simulink model "HDLLTE"  (R2017b)
settings: Solver=FixedStepDiscrete  StartTime=0.0  StopTime=simParams.stopTime  RelTol=1e-3
InitFcn:
  | simParams = hdlcoder_lteofdm_modDetectref_init;
  | simParams = hdlcoder_lteofdm_modDetecthdl_init(simParams);
StopFcn:
  | hdlcoder_lteofdm_modDetect_analyze;
undefined symbols (not defined in the file): fft_size
libraries: hdlsllib x29, simulink x22, simulink_need_slupdate x13, dspxfrm3 x2, commchan3 x1, dspmlti4 x1, commrflib2 x1, hdlcodermisc x1, dspsigops x1, dspmathops x1, dspsrcs4 x1
(part 1 of 3)
CloseFcn:
  | if exist('fig', 'var')
  | 
  |     if ishandle(fig.SSS)
  |         close(fig.SSS);
  |     end
  | 
  |     if ishandle(fig.PSS)
  |         close(fig.PSS);
  |     end
  | 
  |     if ishandle(fig.FRQEST)
  |         close(fig.FRQEST);
  |     end
  | 
  |     if ishandle(fig.TX)
  |         close(fig.TX);
  |     end
  | 
  |     if ishandle(fig.Text)
  |         close(fig.Text);
  |     end
  | 
  |     clear CellID correlationOutput;
  |     clear pCellID sCellID PSSpeak PSStimingOffset fig;
  |     clear simLTERxData simLTERxDataValid;
  |     clear simLTETxData simLTETxDataValid;
  |     clear simParams thresholdOut;
  |     clear primaryCellID;
  | 
  | end
settings Model: DataTypeOverride=Off  Creator=The MathWorks, Inc.  LastModifiedBy=trainee
settings DataIOCC: LimitDataPoints=on  SaveFormat=Array  SaveOutput=off  VisualizeSimOutput=off  SaveTime=off
settings OptimizationCC: BlockReduction=off  BooleanDataType=off  ConditionallyExecuteInputs=off  DefaultParameterBehavior=Inlined  LifeSpan=inf
settings DebuggingCC: AlgebraicLoopMsg=error  SaveWithParameterizedLinksMsg=none  UnderspecifiedInitializationDetection=Classic  MergeDetectMultiDrivingBlocksExec=none  SignalResolutionControl=TryResolveAllWithWarning  SingleTaskRateTransMsg=error  ParameterPrecisionLossMsg=none  AllowSymbolicDim=off  StrictBusMsg=ErrorOnBusTreatedAsVector  SFUnexpectedBacktrackingDiag=warning  SFNoUnconditionalDefaultTransitionDiag=warning  SFExecutionAtInitializationDiag=none
settings HardwareCC: ProdBitPerPointer=32  ProdBitPerSizeT=32  ProdBitPerPtrDiffT=32  ProdLargestAtomicFloat=None  ProdIntDivRoundTo=Undefined  ProdEndianess=Unspecified  ProdWordSize=32  ProdHWDeviceType=ASIC/FPGA->ASIC/FPGA  TargetBitPerPointer=64  TargetBitPerSizeT=64  TargetBitPerPtrDiffT=64  TargetLongLongMode=on  TargetIntDivRoundTo=Zero  TargetEndianess=LittleEndian  TargetWordSize=64  TargetHWDeviceType=MATLAB Host  ProdEqTarget=off
settings ModelReferenceCC: PropagateSignalLabelsOutOfModel=off
settings CodeAppCC: StateflowObjectComments=on
settings GRTTargetCC: TargetLangStandard=C89/C90 (ANSI)  GeneratePreprocessorConditionals=Disable all
settings ConfigComp: CovMetricSettings=dw  CovHtmlReporting=on  CovSaveCumulativeToWorkspaceVar=on  CovSaveSingleToWorkspaceVar=on  CovExternalEMLEnable=off  CovSFcnEnable=off

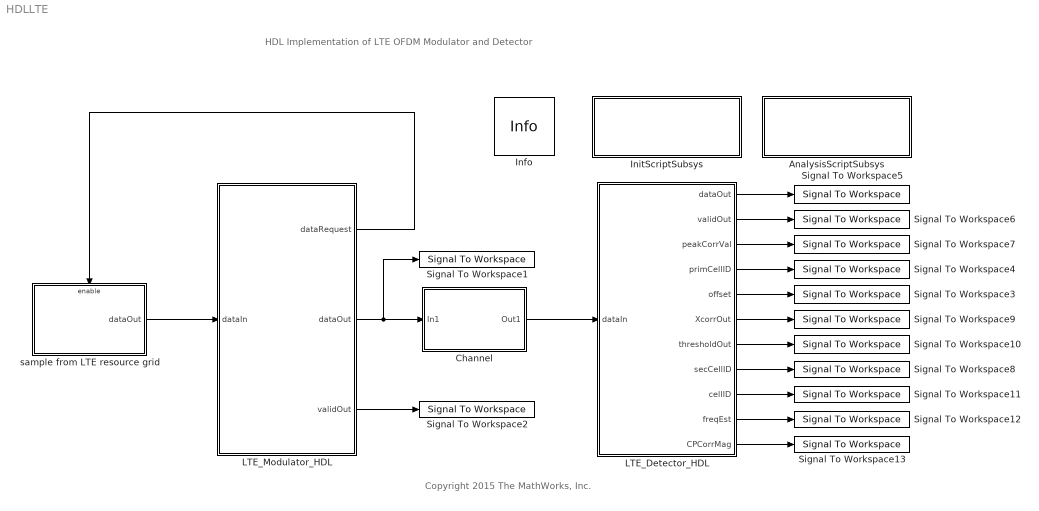
== system HDLLTE ==
  note: HDL Implementation of LTE OFDM Modulator and Detector
  note: Copyright 2015 The MathWorks, Inc.
  AnalysisScriptSubsys : Subsystem
      settings: OpenFcn=edit hdlcoder_lteofdm_modDetect_analyze;
      mask Display: disp('Open post-simulation\n analysis script');
  Channel : Subsystem  mask{timeDelay=simParams.channelDelay, SNR=simParams.channelSNR, gain=simParams.channelGain, frequency=simParams.frequencyOffset}
      mask prompts: timeDelay "Time Delay (samples)"; SNR "SNR (dB)"; gain "Channel Gain"; frequency "Frequency Offset (Hz)"
      mask Display: disp('AWGN &\nFrequency Offset')
  Info : hdlcodermisc/Info  SystemSampleTime=-1
      settings: SourceProductName=HDL Coder  SourceProductBaseCode=HD
  InitScriptSubsys : Subsystem
      settings: OpenFcn=edit hdlcoder_lteofdm_modDetectref_init;
      mask Display: disp('Open LTE initialization\nscript');
  LTE_Detector_HDL : Subsystem
  LTE_Modulator_HDL : Subsystem
  Signal To Workspace1 : SignalToWorkspace  VariableName=simLTETxData
      settings: CopyFcn=dspblkcopystw(gcbh);
  Signal To Workspace10 : SignalToWorkspace  VariableName=thresholdOut
      settings: CopyFcn=dspblkcopystw(gcbh);
  Signal To Workspace11 : SignalToWorkspace  VariableName=cellID
      settings: CopyFcn=dspblkcopystw(gcbh);
  Signal To Workspace12 : SignalToWorkspace  VariableName=freqEst
      settings: CopyFcn=dspblkcopystw(gcbh);
  Signal To Workspace13 : SignalToWorkspace  VariableName=CPCorrMag
      settings: CopyFcn=dspblkcopystw(gcbh);
  Signal To Workspace2 : SignalToWorkspace  VariableName=simLTETxDataValid
      settings: CopyFcn=dspblkcopystw(gcbh);
  Signal To Workspace3 : SignalToWorkspace  VariableName=timingOffset
      settings: CopyFcn=dspblkcopystw(gcbh);
  Signal To Workspace4 : SignalToWorkspace  VariableName=primaryCellID
      settings: CopyFcn=dspblkcopystw(gcbh);
  Signal To Workspace5 : SignalToWorkspace  VariableName=simLTERxData
      settings: CopyFcn=dspblkcopystw(gcbh);
  Signal To Workspace6 : SignalToWorkspace  VariableName=simLTERxDataValid
      settings: CopyFcn=dspblkcopystw(gcbh);
  Signal To Workspace7 : SignalToWorkspace  VariableName=peakCorrelationOutput
      settings: CopyFcn=dspblkcopystw(gcbh);
  Signal To Workspace8 : SignalToWorkspace  VariableName=secondaryCellID
      settings: CopyFcn=dspblkcopystw(gcbh);
  Signal To Workspace9 : SignalToWorkspace  VariableName=correlationOutput
      settings: CopyFcn=dspblkcopystw(gcbh);
  sample from LTE resource grid : Subsystem
  wires:
  LTE_Modulator_HDL/2(dataOut) -> Signal To Workspace1/1, Channel/1(In1)
  LTE_Modulator_HDL/1(dataRequest) -> sample from LTE resource grid/Enable
  sample from LTE resource grid/1(dataOut) -> LTE_Modulator_HDL/1(dataIn)
  LTE_Detector_HDL/1(dataOut) -> Signal To Workspace5/1
  LTE_Detector_HDL/2(validOut) -> Signal To Workspace6/1
  LTE_Detector_HDL/5(offset) -> Signal To Workspace3/1
  LTE_Detector_HDL/7(thresholdOut) -> Signal To Workspace10/1
  LTE_Detector_HDL/6(XcorrOut) -> Signal To Workspace9/1
  LTE_Detector_HDL/3(peakCorrVal) -> Signal To Workspace7/1
  LTE_Detector_HDL/4(primCellID) -> Signal To Workspace4/1
  Channel/1(Out1) -> LTE_Detector_HDL/1(dataIn)
  LTE_Detector_HDL/8(secCellID) -> Signal To Workspace8/1
  LTE_Detector_HDL/9(cellID) -> Signal To Workspace11/1
  LTE_Modulator_HDL/3(validOut) -> Signal To Workspace2/1
  LTE_Detector_HDL/10(freqEst) -> Signal To Workspace12/1
  LTE_Detector_HDL/11(CPCorrMag) -> Signal To Workspace13/1

== system HDLLTE/AnalysisScriptSubsys ==

== system HDLLTE/Channel ==
  In1 : Inport
  ADC : DataTypeConversion  OutDataTypeStr=fixdt(1,16,14)  RndMeth=Nearest
  AWGN : commchan3/AWGN Channel  InputProcessing=Columns as channels (frame based)  seed=67  noiseMode="Signal to noise ratio  (SNR)"  EbNodB=ebno  EsNodB=10  SNRdB=SNR  bitsPerSym=1  Ps=0.0011  Tsym=1  variance=1
  Channel Attenuation : Gain  Gain=gain
  DAC : DataTypeConversion  OutDataTypeStr=double  RndMeth=Nearest
  FIR Decimation : dspmlti4/FIR Decimation  FilterSource=Dialog parameters  h=simParams.hm.*simParams.m  D=simParams.m  filtStruct=Direct form  FilterObject=Hm_firdecim  framing=Allow multirate processing  inputOffset=0  outputBufInitCond=0  roundingMode=Floor  overflowMode=off  firstCoeffDataTypeStr=Inherit: Same word length as input  firstCoeffMin=[]  firstCoeffMax=[]  firstCoeffLastDataTypeStr=Inherit: Same word length as input  outputMin=[]  outputMax=[]
  Phase/ Frequency Offset : commrflib2/Phase// Frequency Offset  phaseOffset=0  freqPort=off  freqOffset=frequency
      settings: SourceProductName=Communications System Toolbox
  Time Delay : Delay  DelayLength=timeDelay  InitialCondition=0
  Out1 : Outport
  wires:
  In1/1 -> DAC/1
  AWGN/1 -> Time Delay/1
  ADC/1 -> Out1/1
  Channel Attenuation/1 -> Phase/ Frequency Offset/1
  Time Delay/1 -> Channel Attenuation/1
  FIR Decimation/1 -> ADC/1
  DAC/1 -> AWGN/1
  Phase/ Frequency Offset/1 -> FIR Decimation/1

== system HDLLTE/InitScriptSubsys ==

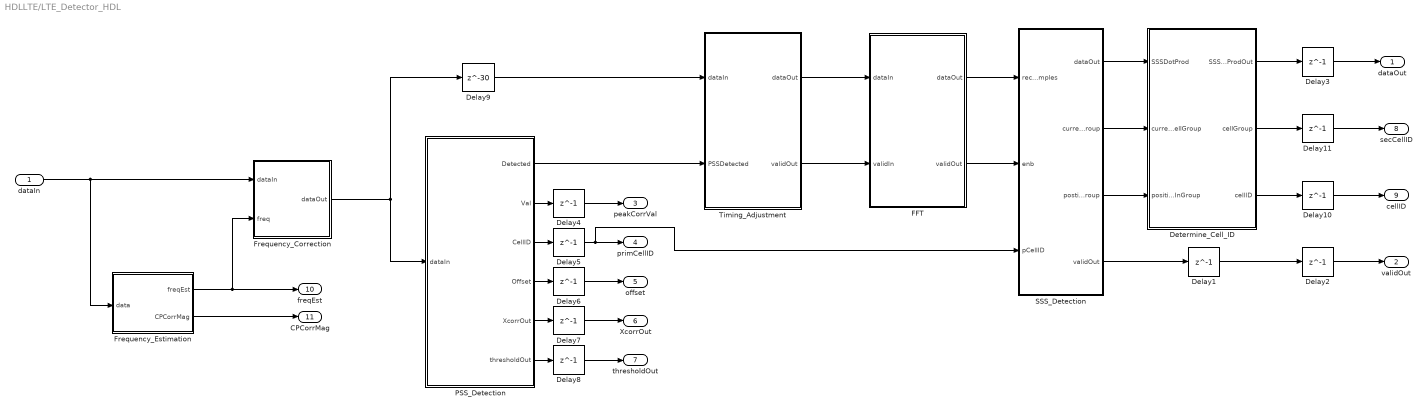
== system HDLLTE/LTE_Detector_HDL ==
  dataIn : Inport
  Delay{1..8,10..11} (10 alike) : Delay  DelayLength=1  InitialCondition=0  UseCircularBuffer=on
  Delay9 : Delay  DelayLength=30  InitialCondition=0  InputProcessing=Columns as channels (frame based)
  Determine_Cell_ID : Subsystem
  FFT : Subsystem
  Frequency_Correction : Subsystem
  Frequency_Estimation : Subsystem
  PSS_Detection : Subsystem
  SSS_Detection : Subsystem
  Timing_Adjustment : Subsystem
  dataOut : Outport
  validOut : Outport  Port=2
  peakCorrVal : Outport  Port=3
  primCellID : Outport  Port=4
  offset : Outport  Port=5
  XcorrOut : Outport  Port=6
  thresholdOut : Outport  Port=7
  secCellID : Outport  Port=8
  cellID : Outport  Port=9
  freqEst : Outport  Port=10
  CPCorrMag : Outport  Port=11
  wires:
  Timing_Adjustment/2(validOut) -> FFT/2(validIn)
  FFT/2(validOut) -> SSS_Detection/2(enb)
  Delay9/1 -> Timing_Adjustment/1(dataIn)
  FFT/1(dataOut) -> SSS_Detection/1(receiveSamples)
  Timing_Adjustment/1(dataOut) -> FFT/1(dataIn)
  SSS_Detection/1(dataOut) -> Determine_Cell_ID/1(SSSDotProd)
  SSS_Detection/2(currentCellGroup) -> Determine_Cell_ID/2(currentCellGroup)
  SSS_Detection/3(postionInGroup) -> Determine_Cell_ID/3(positionInGroup)
  Determine_Cell_ID/1(SSSDotProdOut) -> Delay3/1
  Determine_Cell_ID/2(cellGroup) -> Delay11/1
  Determine_Cell_ID/3(cellID) -> Delay10/1
  SSS_Detection/4(validOut) -> Delay1/1
  Delay1/1 -> Delay2/1
  Delay3/1 -> dataOut/1
  Delay2/1 -> validOut/1
  PSS_Detection/2(Val) -> Delay4/1
  Delay4/1 -> peakCorrVal/1
  PSS_Detection/3(CellID) -> Delay5/1
  Delay5/1 -> SSS_Detection/3(pCellID), primCellID/1
  PSS_Detection/4("Offset ") -> Delay6/1
  Delay6/1 -> offset/1
  PSS_Detection/5(XcorrOut) -> Delay7/1
  Delay7/1 -> XcorrOut/1
  PSS_Detection/6(thresholdOut) -> Delay8/1
  Delay8/1 -> thresholdOut/1
  Delay11/1 -> secCellID/1
  Delay10/1 -> cellID/1
  PSS_Detection/1(Detected) -> Timing_Adjustment/2(PSSDetected)
  dataIn/1 -> Frequency_Estimation/1(data), Frequency_Correction/1(dataIn)
  Frequency_Correction/1(dataOut) -> PSS_Detection/1(dataIn), Delay9/1
  Frequency_Estimation/2(CPCorrMag) -> CPCorrMag/1
  Frequency_Estimation/1(freqEst) -> Frequency_Correction/2(freq), freqEst/1

== system HDLLTE/LTE_Modulator_HDL ==
  dataIn : Inport
  CP_Extension_Windowing : Subsystem
  Delay2 : Delay  DelayLength=1  InitialCondition=0  InputProcessing=Columns as channels (frame based)
  Delay3 : Delay  DelayLength=1
  Delay4 : Delay  DelayLength=1
  Delay5 : Delay
  Delay6 : Delay  DelayLength=1
  FFT_Shift : Subsystem
  Filtering : Subsystem
  IFFT : Subsystem
  OFDM_Symbol_Mapping : Subsystem
  dataRequest : Outport
  dataOut : Outport  Port=2
  validOut : Outport  Port=3
  wires:
  dataIn/1 -> Delay2/1
  OFDM_Symbol_Mapping/1(dataRequest) -> Delay4/1
  OFDM_Symbol_Mapping/3(validOut) -> FFT_Shift/2(validIn)
  OFDM_Symbol_Mapping/2(dataOut) -> FFT_Shift/1(dataIn)
  FFT_Shift/2(validOut) -> IFFT/2(validIn)
  FFT_Shift/1(dataOut) -> IFFT/1(dataIn)
  IFFT/1(dataOut) -> CP_Extension_Windowing/1(dataIn)
  IFFT/2(validOut) -> CP_Extension_Windowing/2(validIn)
  CP_Extension_Windowing/1(dataOut) -> Filtering/1(dataIn)
  Filtering/1(dataOut) -> Delay3/1
  Delay2/1 -> OFDM_Symbol_Mapping/1(dataIn)
  Delay3/1 -> dataOut/1
  Delay4/1 -> dataRequest/1
  CP_Extension_Windowing/2(validOut) -> Delay5/1
  Delay5/1 -> Delay6/1
  Delay6/1 -> validOut/1

== system HDLLTE/sample from LTE resource grid ==
  request1 : EnablePort
  Data Type Conversion : DataTypeConversion  OutDataTypeStr=fixdt(1,16,14)  RndMeth=Nearest
  sample from LTE resource grid : dspsrcs4/Signal From Workspace  X=simParams.LTEGrid(:)  Ts=simParams.TsTx  nsamps=1  OutputAfterFinalValue=Setting to zero  ignoreOrWarnInputAndFrameLengths=off  OutputFrames=on
  dataOut : Outport
  wires:
  Data Type Conversion/1 -> dataOut/1
  sample from LTE resource grid/1 -> Data Type Conversion/1

== system HDLLTE/LTE_Detector_HDL/Determine_Cell_ID ==
  note: N_ID(2)
  note: Calculate detected Cell ID
      | (CellID = 3*N_ID(1) + N_ID(2))
  note: N_ID(1)
  note: If incoming SSS correlation output is greater than that stored in register,
      | store new maximum value, and cell group number, in registers
  note: Store maximum value in register
  note: Store corresponding cell group in register
  SSSDotProd : Inport
  currentCellGroup : Inport  Port=2
  positionInGroup : Inport  Port=3
  Add2 : Sum  OutDataTypeStr=Inherit: Same as first input
  Delay10 : Delay  DelayLength=1  InitialCondition=0  UseCircularBuffer=on
  Gain1 : Gain  Gain=3  OutDataTypeStr=fixdt(0,9,0)
  Relational Operator4 : RelationalOperator  Operator=>  OutDataTypeStr=boolean  RndMeth=Nearest
  Unit Delay Enabled1 : simulink_need_slupdate/Unit Delay Enabled  vinit=0  tsamp=-1
      settings: SourceProductName=Simulink  SourceProductBaseCode=SL
  Unit Delay Enabled3 : simulink_need_slupdate/Unit Delay Enabled  vinit=0  tsamp=-1
      settings: SourceProductName=Simulink  SourceProductBaseCode=SL
  SSSDotProdOut : Outport
  cellGroup : Outport  Port=2
  cellID : Outport  Port=3
  wires:
  Delay10/1 -> SSSDotProdOut/1
  Add2/1 -> cellID/1
  SSSDotProd/1 -> Unit Delay Enabled3/1, Relational Operator4/1, Delay10/1
  positionInGroup/1 -> Add2/2
  Unit Delay Enabled1/1 -> Gain1/1, cellGroup/1
  currentCellGroup/1 -> Unit Delay Enabled1/1
  Relational Operator4/1 -> Unit Delay Enabled3/2, Unit Delay Enabled1/2
  Gain1/1 -> Add2/1
  Unit Delay Enabled3/1 -> Relational Operator4/2

== system HDLLTE/LTE_Detector_HDL/FFT ==
  note: Set input of FFT to input wordlength + FFT growth to allow
      | the output of the FFT to scale. Maximum bit growth is equal
      | to log2(nFFT).
  dataIn : Inport
  validIn : Inport  Port=2
  Data Type Conversion : DataTypeConversion  OutDataTypeStr=fixdt(1,18,10)  RndMeth=Round
  Delay{1..2,4..5} (4 alike) : Delay  DelayLength=1  InitialCondition=0  InputProcessing=Columns as channels (frame based)
  FFT HDL Optimized : dspxfrm3/FFT HDL Optimized  FFTLength=128  Architecture=Streaming Radix 2^2  ComplexMultiplication=Use 3 multipliers and 5 adders  BitReversedOutput=off  BitReversedInput=off  Normalize=off  SimulateUsing=Code generation  RoundingMethod=Floor  ResetInputPort=off  StartOutputPort=off  EndOutputPort=off
      settings: SourceProductName=DSP System Toolbox  SourceProductBaseCode=DS
  Signal Specification : SignalSpecification  Dimensions=1
  Signal Specification1 : SignalSpecification  Dimensions=1
  dataOut : Outport
  validOut : Outport  Port=2
  wires:
  Signal Specification1/1 -> FFT HDL Optimized/2
  Signal Specification/1 -> FFT HDL Optimized/1
  FFT HDL Optimized/2 -> Delay5/1
  FFT HDL Optimized/1 -> Delay4/1
  Delay4/1 -> Data Type Conversion/1
  Delay2/1 -> Signal Specification1/1
  dataIn/1 -> Delay1/1
  validIn/1 -> Delay2/1
  Delay1/1 -> Signal Specification/1
  Data Type Conversion/1 -> dataOut/1
  Delay5/1 -> validOut/1

== system HDLLTE/LTE_Detector_HDL/Frequency_Correction ==
  note: This subsystem corrects the frequency offset using an Numerically Controller Oscillator (NCO) and a conjugate multiplication.
  dataIn : Inport
  freq : Inport  Port=2
  Data Type Conversion : DataTypeConversion  OutDataTypeStr=fixdt(1,16,15)  RndMeth=Nearest
  Delay{1..6} (6 alike) : Delay  DelayLength=1  InitialCondition=0  UseCircularBuffer=on
  Gain : Gain  Gain=2^9  OutDataTypeStr=int16
  NCO HDL Optimized : dspsigops/NCO HDL Optimized  PhaseIncrementSource=Input port  PhaseIncrement=100  PhaseOffsetSource=Property  PhaseOffset=0  DitherSource=Property  NumDitherBits=4  PhaseQuantization=on  NumQuantizerAccumulatorBits=12  LUTCompress=on  ResetAction=off  ValidInputPort=off  Waveform=Complex exponential  PhasePort=off  SimulateUsing=Code generation  AccumulatorWL=16  OutputDataType=Binary point scaling  OutputWL=16  OutputFL=14
      settings: SourceProductName=DSP System Toolbox  SourceProductBaseCode=DS
  Product1 : Product
  Signal Spec : SignalSpecification  Dimensions=1
  Unit Delay Enabled : simulink_need_slupdate/Unit Delay Enabled  vinit=0.0  tsamp=-1
      settings: SourceProductName=Simulink  SourceProductBaseCode=SL
  complexConjugate : Math  Operator=conj  SaturateOnIntegerOverflow=on
  dataOut : Outport
  wires:
  complexConjugate/1 -> Delay3/1
  NCO HDL Optimized/2 -> Unit Delay Enabled/2
  dataIn/1 -> Delay2/1
  Product1/1 -> Delay4/1
  NCO HDL Optimized/1 -> Unit Delay Enabled/1
  Unit Delay Enabled/1 -> complexConjugate/1
  Data Type Conversion/1 -> Delay1/1
  Delay2/1 -> Product1/1
  Delay1/1 -> dataOut/1
  Delay4/1 -> Data Type Conversion/1
  Delay3/1 -> Product1/2
  Gain/1 -> Delay5/1
  freq/1 -> Delay6/1
  Delay6/1 -> Gain/1
  Signal Spec/1 -> NCO HDL Optimized/1
  Delay5/1 -> Signal Spec/1

== system HDLLTE/LTE_Detector_HDL/Frequency_Estimation ==
  data : Inport
  Angle_Filter : Subsystem
  Angle_at_Maximum : Subsystem
  Cyclic_Prefix_Correlator : Subsystem
  Rect_to_Polar : Subsystem
  freqEst : Outport
  CPCorrMag : Outport  Port=2
  wires:
  data/1 -> Cyclic_Prefix_Correlator/1(dataIn)
  Rect_to_Polar/3(validOut) -> Angle_at_Maximum/3(validIn)
  Angle_at_Maximum/1(angleOut) -> Angle_Filter/1(angleIn)
  Rect_to_Polar/2(angleOut) -> Angle_at_Maximum/2(angleIn)
  Rect_to_Polar/1(magOut) -> CPCorrMag/1, Angle_at_Maximum/1(magIn)
  Cyclic_Prefix_Correlator/1(corrOut) -> Rect_to_Polar/1(dataIn)
  Angle_Filter/1(angleOut) -> freqEst/1
  Angle_at_Maximum/2(validOut) -> Angle_Filter/2(en)

== system HDLLTE/LTE_Detector_HDL/PSS_Detection ==
  dataIn : Inport
  Cross_Correlation : Subsystem
  Delay4 : Delay  DelayLength=4  InitialCondition=0  InputProcessing=Columns as channels (frame based)
  Determine_Primary_Cell_ID : Subsystem
  Peak_Detection : Subsystem
  Detected : Outport
  Val : Outport  Port=2
  CellID : Outport  Port=3
  "Offset " : Outport  Port=4
  XcorrOut : Outport  Port=5
  thresholdOut : Outport  Port=6  InitialOutput=0
  wires:
  Determine_Primary_Cell_ID/1(Val) -> Val/1
  Determine_Primary_Cell_ID/2(Cell_ID) -> CellID/1
  Determine_Primary_Cell_ID/4(PSSDetected) -> Detected/1
  Determine_Primary_Cell_ID/3("Offset ") -> "Offset "/1
  Determine_Primary_Cell_ID/5(XcorrOut) -> XcorrOut/1
  Delay4/1 -> thresholdOut/1
  Cross_Correlation/1(PSS0) -> Peak_Detection/1(PSS0)
  Cross_Correlation/2(PSS1) -> Peak_Detection/2(PSS1)
  Cross_Correlation/3(PSS2) -> Peak_Detection/3(PSS2)
  Cross_Correlation/4(Threshold) -> Peak_Detection/4(thresholdIn)
  Peak_Detection/4(PSS0Strength) -> Determine_Primary_Cell_ID/3(PSS0Strength)
  Peak_Detection/12(Xcorr1Out) -> Determine_Primary_Cell_ID/11(Xcorr1In)
  Peak_Detection/7(PSS1Strength) -> Determine_Primary_Cell_ID/6(PSS1Strength)
  Peak_Detection/8(PSS2Detected) -> Determine_Primary_Cell_ID/7(PSS2Detected)
  Peak_Detection/10(PSS2Strength) -> Determine_Primary_Cell_ID/9(PSS2Strength)
  Peak_Detection/2(PSS0Detected) -> Determine_Primary_Cell_ID/1(PSS0Detected)
  Peak_Detection/6(PSS1Offset) -> Determine_Primary_Cell_ID/5(PSS1Offset)
  Peak_Detection/3(PSS0Offset) -> Determine_Primary_Cell_ID/2(PSS0Offset)
  Peak_Detection/9(PSS2Offset) -> Determine_Primary_Cell_ID/8(PSS2Offset)
  Peak_Detection/5(PSS1Detected) -> Determine_Primary_Cell_ID/4(PSS1Detected)
  Peak_Detection/11(Xcorr0Out) -> Determine_Primary_Cell_ID/10(Xcorr0In)
  Peak_Detection/13(Xcorr2Out) -> Determine_Primary_Cell_ID/12(Xcorr2In)
  Peak_Detection/1(thresholdOut) -> Delay4/1
  dataIn/1 -> Cross_Correlation/1(dataIn)

== system HDLLTE/LTE_Detector_HDL/SSS_Detection ==
  receiveSamples : Inport
  enb : Inport  Port=2
  pCellID : Inport  Port=3
  Delay1 : Delay  DelayLength=8  InitialCondition=0  UseCircularBuffer=on
  Delay{2,4..7,9..10} (7 alike) : Delay  DelayLength=1  InitialCondition=0  UseCircularBuffer=on
  Delay11 : Delay  DelayLength=4  InitialCondition=0
  Delay12 : Delay  DelayLength=4  InitialCondition=0
  Delay3 : Delay  InitialCondition=0
  Delay8 : Delay  DelayLength=8  InitialCondition=0  UseCircularBuffer=on
  SSS_Dot_Product : Subsystem
  SSS_Sequence_Update : Subsystem
  Sample_and_Store : Subsystem
  dataOut : Outport
  currentCellGroup : Outport  Port=2
  postionInGroup : Outport  Port=3
  validOut : Outport  Port=4
  wires:
  SSS_Dot_Product/2(SSSDotProd) -> Delay4/1
  SSS_Dot_Product/1(validOut) -> Delay9/1
  Delay3/1 -> SSS_Sequence_Update/3(PositionInGroup)
  Sample_and_Store/3(groupCount) -> SSS_Sequence_Update/2(cellGroup)
  Delay2/1 -> Delay3/1
  enb/1 -> Delay6/1
  receiveSamples/1 -> Delay7/1
  pCellID/1 -> Delay2/1
  Sample_and_Store/2(validOut) -> SSS_Sequence_Update/1(validIn)
  Delay7/1 -> Sample_and_Store/1(samplesIn)
  Delay6/1 -> Sample_and_Store/2(enb)
  Sample_and_Store/1(dataOut) -> Delay12/1
  SSS_Sequence_Update/1(validOut) -> SSS_Dot_Product/2(validIn)
  SSS_Sequence_Update/2(seqOut) -> SSS_Dot_Product/3(seqIn)
  SSS_Sequence_Update/3(endofGroup) -> SSS_Dot_Product/4(reset)
  SSS_Sequence_Update/4(detectedPSS) -> Delay8/1
  Delay8/1 -> Delay10/1
  Delay1/1 -> Delay5/1
  Delay10/1 -> postionInGroup/1
  Delay5/1 -> currentCellGroup/1
  Delay4/1 -> dataOut/1
  Delay9/1 -> validOut/1
  Sample_and_Store/4(currentCellGroup) -> Delay11/1
  Delay11/1 -> Delay1/1
  Delay12/1 -> SSS_Dot_Product/1(dataIn)

== system HDLLTE/LTE_Detector_HDL/Timing_Adjustment ==
  note: Detect PSS detection strobe, and create
      | valid high signal.
  note: Delay signal so that once the PSS
      | has been detected, the resource block
      | containing the SSS signal (the previous
      | block) is aligned here.
  note: Only output samples once
      | the detected strobe has
      | been received.
  note: PSS detect strobe is high at the end of the PSS
      | sequence, so delay must be for the full 128 samples
      | of the PSS, and the full 128 samples of the SSS, plus
      | a single short CP length of 9 samples for 128-point
      | FFT.
  dataIn : Inport
  PSSDetected : Inport  Port=2
  Constant : Constant  Value=complex(0)  OutDataTypeStr=fixdt(1,16,15)  SampleTime=simParams.TsRx
  Constant1 : Constant  OutDataTypeStr=boolean  SampleTime=simParams.TsRx
  Delay1 : Delay  DelayLength=265  InitialCondition=0  InputProcessing=Columns as channels (frame based)
  Delay{2..5} (4 alike) : Delay  DelayLength=1  InitialCondition=0  UseCircularBuffer=on
  Switch : Switch  Criteria=u2 > Threshold
  Unit Delay Enabled1 : simulink_need_slupdate/Unit Delay Enabled  vinit=0.0  tsamp=-1
      settings: SourceProductName=Simulink  SourceProductBaseCode=SL
  dataOut : Outport
  validOut : Outport  Port=2
  wires:
  Delay5/1 -> validOut/1
  Delay4/1 -> dataOut/1
  Delay3/1 -> Delay1/1
  Delay2/1 -> Unit Delay Enabled1/2
  Constant/1 -> Switch/3
  Delay1/1 -> Switch/1
  dataIn/1 -> Delay3/1
  Switch/1 -> Delay4/1
  PSSDetected/1 -> Delay2/1
  Unit Delay Enabled1/1 -> Switch/2, Delay5/1
  Constant1/1 -> Unit Delay Enabled1/1

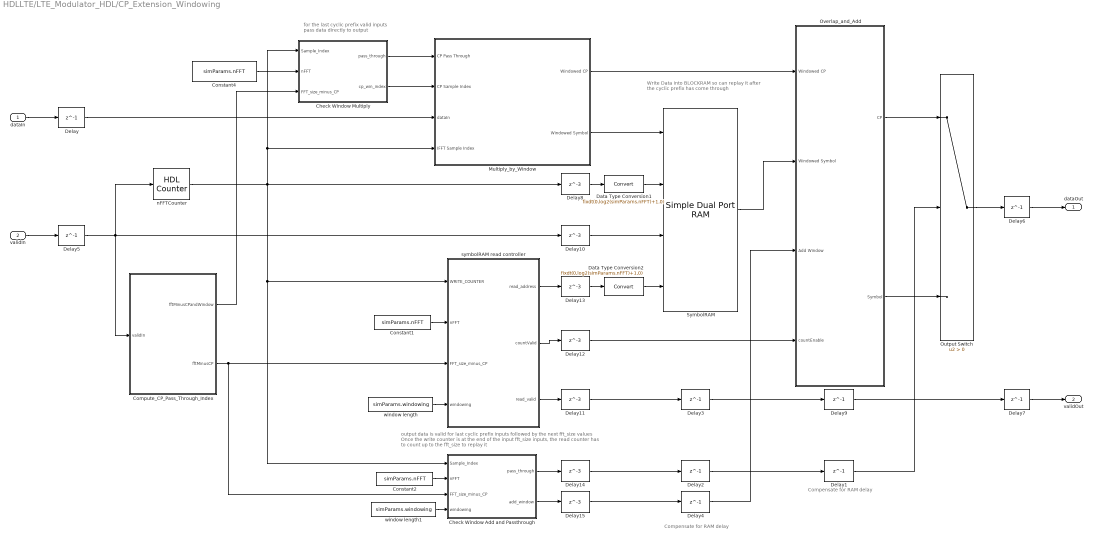
== system HDLLTE/LTE_Modulator_HDL/CP_Extension_Windowing ==
  note: Compensate for RAM delay
  note: output data is valid for last cyclic prefix inputs followed by the next fft_size values
      | Once the write counter is at the end of the input fft_size inputs,
      | the read counter has to count up to the fft_size to replay it
  note: Write Data into BLOCKRAM so can
      | replay it after the cyclic prefix has come through
  note: for the last cyclic prefix valid inputs
      | pass data directly to output
  note: Compensate for RAM delay
  dataIn : Inport
  validIn : Inport  Port=2
  Check Window Add and Passthrough : MATLAB Function  TreatAsAtomicUnit=on
  "Check Window Multiply " : MATLAB Function  TreatAsAtomicUnit=on
  Compute_CP_Pass_Through_Index : Subsystem
  Constant1 : Constant  Value=simParams.nFFT  VectorParams1D=off  OutDataTypeStr=uint16  SampleTime=simParams.TsTx
  Constant2 : Constant  Value=simParams.nFFT  VectorParams1D=off  OutDataTypeStr=uint16  SampleTime=simParams.TsTx
  Constant4 : Constant  Value=simParams.nFFT  VectorParams1D=off  OutDataTypeStr=uint16  SampleTime=simParams.TsTx
  Data Type Conversion1 : DataTypeConversion  OutDataTypeStr=fixdt(0,log2(simParams.nFFT)+1,0)
  Data Type Conversion2 : DataTypeConversion  OutDataTypeStr=fixdt(0,log2(simParams.nFFT)+1,0)
  Delay{,5..7} (4 alike) : Delay  DelayLength=1
  Delay1 : Delay  DelayLength=1  InitialCondition=0  UseCircularBuffer=on
  Delay{8,10..15} (7 alike) : Delay  DelayLength=3  InitialCondition=0  InputProcessing=Columns as channels (frame based)
  Delay2 : Delay  DelayLength=1  InitialCondition=0  InputProcessing=Columns as channels (frame based)
  Delay3 : Delay  DelayLength=1  InitialCondition=0  InputProcessing=Columns as channels (frame based)
  Delay4 : Delay  DelayLength=1  InitialCondition=0  InputProcessing=Columns as channels (frame based)
  Delay9 : Delay  DelayLength=1  InitialCondition=0  UseCircularBuffer=on
  Multiply_by_Window : Subsystem
  Output Switch : Switch  Criteria=u2 > Threshold
  Overlap_and_Add : Subsystem
  SymbolRAM : hdlsllib/HDL RAMs/Simple Dual Port RAM  ram_size=log2(simParams.nFFT)+1
      settings: SourceProductName=HDL Coder  SourceProductBaseCode=HD
  nFFTCounter : hdlsllib/Sources/HDL Counter  CountType=Count limited  CountInit=0  CountStep=1  CountMax=simParams.nFFT-1  CountFromType=Initial value  CountFrom=0  CountResetPort=off  CountLoadPort=off  CountEnbPort=on  CountDirPort=off  CountDataType=Unsigned  CountWordLen=log2(simParams.nFFT)  CountFracLen=0  CountSampTime=1
      settings: SourceProductBaseCode=HD
  symbolRAM read controller : MATLAB Function  TreatAsAtomicUnit=on
  window length : Constant  Value=simParams.windowing  OutDataTypeStr=uint16  SampleTime=simParams.TsTx
  window length1 : Constant  Value=simParams.windowing  OutDataTypeStr=uint16  SampleTime=simParams.TsTx
  dataOut : Outport
  validOut : Outport  Port=2
  wires:
  Data Type Conversion1/1 -> SymbolRAM/2
  Data Type Conversion2/1 -> SymbolRAM/4
  "Check Window Multiply "/1(pass_through) -> Multiply_by_Window/1(CP Pass Through)
  Output Switch/1 -> Delay6/1
  symbolRAM read controller/1(read_address) -> Delay13/1
  Compute_CP_Pass_Through_Index/1(fftMinusCPandWindow) -> "Check Window Multiply "/3(FFT_size_minus_CP)
  validIn/1 -> Delay5/1
  "Check Window Multiply "/2(cp_win_index) -> Multiply_by_Window/2(CP Sample Index)
  dataIn/1 -> Delay/1
  Multiply_by_Window/2(Windowed Symbol) -> SymbolRAM/1
  Compute_CP_Pass_Through_Index/2(fftMinusCP) -> Check Window Add and Passthrough/3(FFT_size_minus_CP), symbolRAM read controller/3(FFT_size_minus_CP)
  SymbolRAM/1 -> Overlap_and_Add/2(Windowed Symbol)
  Delay4/1 -> Overlap_and_Add/3(Add Window)
  Overlap_and_Add/2(Symbol) -> Output Switch/3
  Delay3/1 -> Delay9/1
  Delay9/1 -> Delay7/1
  Delay2/1 -> Delay1/1
  Delay1/1 -> Output Switch/2
  Multiply_by_Window/1(Windowed CP) -> Overlap_and_Add/1(Windowed CP)
  Delay/1 -> Multiply_by_Window/3(dataIn)
  Delay6/1 -> dataOut/1
  Delay7/1 -> validOut/1
  nFFTCounter/1 -> "Check Window Multiply "/1(Sample_Index), Multiply_by_Window/4(IFFT Sample Index), Delay8/1, Check Window Add and Passthrough/1(Sample_Index), symbolRAM read controller/1(WRITE_COUNTER)
  Delay5/1 -> nFFTCounter/1, Compute_CP_Pass_Through_Index/1(validIn), Delay10/1
  symbolRAM read controller/2(countValid) -> Delay12/1
  symbolRAM read controller/3(read_valid) -> Delay11/1
  Check Window Add and Passthrough/1(pass_through) -> Delay14/1
  Check Window Add and Passthrough/2(add_window) -> Delay15/1
  Overlap_and_Add/1(CP) -> Output Switch/1
  Delay8/1 -> Data Type Conversion1/1
  Delay10/1 -> SymbolRAM/3
  Delay12/1 -> Overlap_and_Add/4(countEnable)
  Delay11/1 -> Delay3/1
  Delay13/1 -> Data Type Conversion2/1
  Delay14/1 -> Delay2/1
  Delay15/1 -> Delay4/1
  Constant4/1 -> "Check Window Multiply "/2(nFFT)
  Constant1/1 -> symbolRAM read controller/2(nFFT)
  window length/1 -> symbolRAM read controller/4(windowing)
  window length1/1 -> Check Window Add and Passthrough/4(windowing)
  Constant2/1 -> Check Window Add and Passthrough/2(nFFT)

== system HDLLTE/LTE_Modulator_HDL/FFT_Shift ==
  note: Count 2 full FFT frames
  note: If a full IFFT frame OR 2 full FFT frames have been counted and written into RAM, enable reading from RAM.
  note: Compensate for RAM latency
  dataIn : Inport
  validIn : Inport  Port=2
  " " : simulink/Logic and Bit Operations/Compare To Constant  relop===  const=2*simParams.nFFT-1  OutDataTypeStr=boolean
  " " : simulink/Logic and Bit Operations/Compare To Constant  relop===  const=simParams.nFFT-1  OutDataTypeStr=boolean
  Compute_Read_Address : Subsystem
  Data Type Conversion : DataTypeConversion  OutDataTypeStr=fixdt(0,log2(simParams.nFFT)+1,0)
  Data Type Conversion1 : DataTypeConversion  OutDataTypeStr=fixdt(0,log2(simParams.nFFT)+1,0)
  Delay{,1..4} (5 alike) : Delay  DelayLength=1
  Dual Port RAM : hdlsllib/HDL RAMs/Dual Port RAM  ram_size=log2(simParams.nFFT)+1
      settings: SourceProductName=HDL Coder  SourceProductBaseCode=HD
  HDL Counter : hdlsllib/Sources/HDL Counter  CountType=Count limited  CountInit=0  CountStep=1  CountMax=simParams.nFFT*2-1  CountFromType=Initial value  CountFrom=0  CountResetPort=off  CountLoadPort=off  CountEnbPort=on  CountDirPort=off  CountDataType=Unsigned  CountWordLen=log2(simParams.nFFT)+1  CountFracLen=0  CountSampTime=1
      settings: SourceProductBaseCode=HD
  Logical Operator : Logic  Operator=OR  IconShape=distinctive  AllPortsSameDT=off  OutDataTypeStr=boolean
  Terminator : Terminator
  dataOut : Outport
  validOut : Outport  Port=2
  wires:
  validIn/1 -> Delay3/1
  HDL Counter/1 -> " "/1, " "/1, Data Type Conversion/1
  dataIn/1 -> Delay4/1
  Data Type Conversion1/1 -> Dual Port RAM/4
  Data Type Conversion/1 -> Dual Port RAM/2
  Dual Port RAM/1 -> Terminator/1
  " "/1 -> Logical Operator/1
  " "/1 -> Logical Operator/2
  Dual Port RAM/2 -> Delay2/1
  Logical Operator/1 -> Compute_Read_Address/1(rdEnable)
  Compute_Read_Address/1(rdAddr) -> Data Type Conversion1/1
  Compute_Read_Address/2(rdValid) -> Delay/1
  Delay/1 -> Delay1/1
  Delay1/1 -> validOut/1
  Delay2/1 -> dataOut/1
  Delay3/1 -> Dual Port RAM/3, HDL Counter/1
  Delay4/1 -> Dual Port RAM/1

== system HDLLTE/LTE_Modulator_HDL/Filtering ==
  dataIn : Inport
  Delay : Delay  DelayLength=1
  Delay3 : Delay  DelayLength=1
  Filter1 : DiscreteFir  Tag=BlockMethodSubSystem  FilterStructure=Direct form symmetric  Coefficients=simParams.h  OutDataTypeStr=Inherit: Same as input
  dataOut : Outport
  wires:
  dataIn/1 -> Delay/1
  Delay/1 -> Filter1/1
  Delay3/1 -> dataOut/1
  Filter1/1 -> Delay3/1

== system HDLLTE/LTE_Modulator_HDL/IFFT ==
  note: Set input of FFT to input wordlength + FFT growth to allow
      | the output of the FFT to scale. Maximum bit growth is equal
      | to log2(nFFT).
  dataIn : Inport
  validIn : Inport  Port=2
  Data Type Conversion : DataTypeConversion  OutDataTypeStr=fixdt(1,23,21)  RndMeth=Nearest
  Delay{1..2,4..5} (4 alike) : Delay  DelayLength=1  InitialCondition=0  InputProcessing=Columns as channels (frame based)
  IFFT HDL Optimized : dspxfrm3/IFFT HDL Optimized  FFTLength=simParams.nFFT  Architecture=Streaming Radix 2^2  ComplexMultiplication=Use 3 multipliers and 5 adders  BitReversedOutput=off  BitReversedInput=off  Normalize=on  SimulateUsing=Code generation  RoundingMethod=Floor  ResetInputPort=off  StartOutputPort=off  EndOutputPort=off
      settings: SourceProductName=DSP System Toolbox  SourceProductBaseCode=DS
  Signal Specification : SignalSpecification  Dimensions=1
  Signal Specification1 : SignalSpecification  Dimensions=1
  dataOut : Outport
  validOut : Outport  Port=2
  wires:
  validIn/1 -> Delay2/1
  dataIn/1 -> Delay1/1
  Delay4/1 -> dataOut/1
  Delay5/1 -> validOut/1
  Delay1/1 -> Data Type Conversion/1
  Delay2/1 -> Signal Specification1/1
  IFFT HDL Optimized/1 -> Delay4/1
  IFFT HDL Optimized/2 -> Delay5/1
  Signal Specification/1 -> IFFT HDL Optimized/1
  Signal Specification1/1 -> IFFT HDL Optimized/2
  Data Type Conversion/1 -> Signal Specification/1

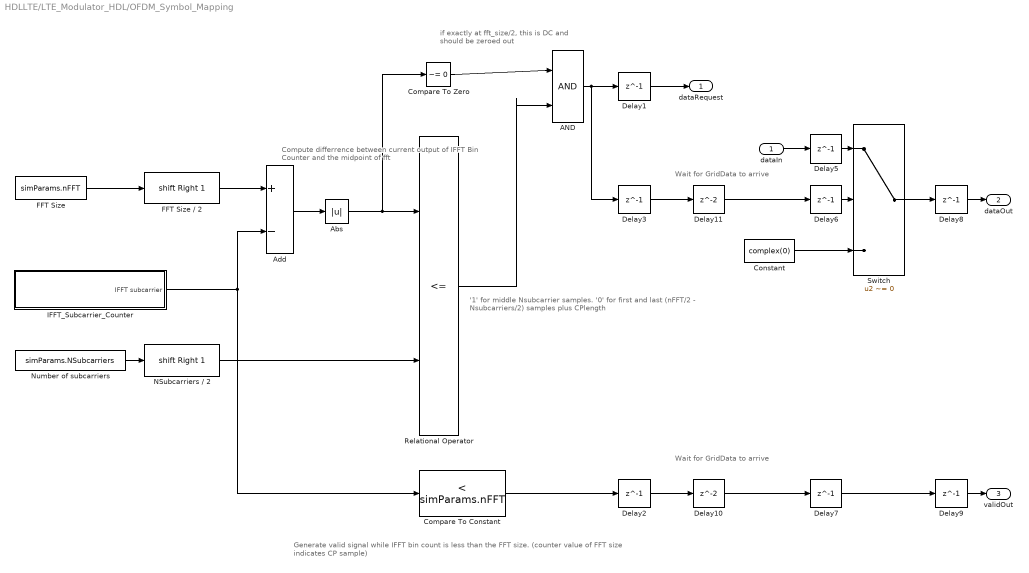
== system HDLLTE/LTE_Modulator_HDL/OFDM_Symbol_Mapping ==
  note: Wait for GridData to
      | arrive
  note: Generate valid signal while IFFT bin count is less than the FFT size.
      | (counter value of FFT size indicates CP sample)
  note: Compute differrence between current output of IFFT Bin Counter and the midpoint of fft
  note: if exactly at fft_size/2, this is DC
      | and should be zeroed out
  note: '1' for middle Nsubcarrier samples.
      | '0' for first and last (nFFT/2 - Nsubcarriers/2) samples
      | plus CPlength
  note: Wait for GridData to
      | arrive
  dataIn : Inport
  AND : Logic  IconShape=distinctive  AllPortsSameDT=off  OutDataTypeStr=boolean
  Abs : Abs
  Add : Sum  Inputs=+-  OutDataTypeStr=fixdt(1,16,0)
  Compare To Constant : simulink/Logic and Bit Operations/Compare To Constant  relop=<  const=simParams.nFFT  OutDataTypeStr=boolean
  Compare To Zero : simulink/Logic and Bit Operations/Compare To Zero  relop=~=  OutDataTypeStr=boolean
  Constant : Constant  Value=complex(0)  OutDataTypeStr=fixdt(1,16,14)  SampleTime=simParams.TsTx
  Delay{1..3,5..9} (8 alike) : Delay  DelayLength=1  InitialCondition=0  InputProcessing=Columns as channels (frame based)
  Delay10 : Delay  InitialCondition=0  InputProcessing=Columns as channels (frame based)
  Delay11 : Delay  InitialCondition=0  InputProcessing=Columns as channels (frame based)
  FFT Size : Constant  Value=simParams.nFFT  OutDataTypeStr=fixdt(0,ceil(log2(simParams.nFFT))+1,0)  SampleTime=simParams.TsTx
  FFT Size / 2 : ArithShift  BitShiftNumber=1  BitShiftDirection=Right
  IFFT_Subcarrier_Counter : Subsystem
  NSubcarriers / 2 : ArithShift  BitShiftNumber=1  BitShiftDirection=Right
  Number of subcarriers : Constant  Value=simParams.NSubcarriers  OutDataTypeStr=fixdt(0,12,0)  SampleTime=simParams.TsTx
  Relational Operator : RelationalOperator  Operator=<=  OutDataTypeStr=boolean  RndMeth=Nearest
  Switch : Switch  Criteria=u2 ~= 0
  dataRequest : Outport
  dataOut : Outport  Port=2
  validOut : Outport  Port=3
  wires:
  Compare To Zero/1 -> AND/1
  Compare To Constant/1 -> Delay2/1
  dataIn/1 -> Delay5/1
  AND/1 -> Delay3/1, Delay1/1
  IFFT_Subcarrier_Counter/1(IFFT subcarrier) -> Add/2, Compare To Constant/1
  FFT Size/1 -> FFT Size / 2/1
  Abs/1 -> Compare To Zero/1, Relational Operator/1
  NSubcarriers / 2/1 -> Relational Operator/2
  Add/1 -> Abs/1
  FFT Size / 2/1 -> Add/1
  Switch/1 -> Delay8/1
  Relational Operator/1 -> AND/2
  Delay2/1 -> Delay10/1
  Delay3/1 -> Delay11/1
  Delay5/1 -> Switch/1
  Constant/1 -> Switch/3
  Delay7/1 -> Delay9/1
  Delay8/1 -> dataOut/1
  Delay9/1 -> validOut/1
  Delay10/1 -> Delay7/1
  Delay11/1 -> Delay6/1
  Delay6/1 -> Switch/2
  Delay1/1 -> dataRequest/1
  Number of subcarriers/1 -> NSubcarriers / 2/1

== system HDLLTE/LTE_Detector_HDL/Frequency_Estimation/Angle_Filter ==
  note: This subsystem implements a 1-pole IIR filter to perform further averaging of the correlation angle results. The filter's gain is normalized to 0dB and an efficient implementation which requires only 1 multiplier is used.
  angleIn : Inport
  en : Inport  Port=2
  Add : Sum  Inputs=|-+
  Add1 : Sum  Inputs=|-+
  Delay1 : Delay  DelayLength=1  InitialCondition=0  UseCircularBuffer=on
  Delay2 : Delay  DelayLength=1  InitialCondition=0  UseCircularBuffer=on
  Delay3 : Delay  DelayLength=1  InitialCondition=0  UseCircularBuffer=on
  Gain : Gain  Gain=2^-2  OutDataTypeStr=Inherit: Same as input
  Unit Delay Enabled : simulink_need_slupdate/Unit Delay Enabled  vinit=0.0  tsamp=-1
      settings: SourceProductName=Simulink  SourceProductBaseCode=SL
  angleOut : Outport
  wires:
  angleIn/1 -> Delay2/1
  Add/1 -> Gain/1
  Gain/1 -> Add1/1
  Unit Delay Enabled/1 -> Add/2, Add1/2, Delay1/1
  Add1/1 -> Unit Delay Enabled/1
  en/1 -> Delay3/1
  Delay1/1 -> angleOut/1
  Delay2/1 -> Add/1
  Delay3/1 -> Unit Delay Enabled/2

== system HDLLTE/LTE_Detector_HDL/Frequency_Estimation/Angle_at_Maximum ==
  note: This subsystem records the maximum CP correlation level, and the corresponding phase angle of the result, across windows of time equivalent to 1 slot (960 samples). A counter is used to reset the running max and record the final phase value, which is then passed to the output and qualified by the validOut signal.
  note: Store current mag & angle if mag is greater than previous max mag.
  note: This register stores the current running max magnitude in the current time window
  magIn : Inport
  angleIn : Inport  Port=2
  validIn : Inport  Port=3
  Compare To Constant : simulink/Logic and Bit Operations/Compare To Constant  relop===  const=0  OutDataTypeStr=boolean
  Delay{1..3,5} (4 alike) : Delay  DelayLength=1  InitialCondition=0  UseCircularBuffer=on
  HDL Counter : hdlsllib/Sources/HDL Counter  CountType=Count limited  CountInit=0  CountStep=1  CountMax=959  CountFromType=Initial value  CountFrom=0  CountResetPort=off  CountLoadPort=off  CountEnbPort=on  CountDirPort=off  CountDataType=Unsigned  CountWordLen=10  CountFracLen=0  CountSampTime=1
      settings: SourceProductBaseCode=HD
  Logical Operator : Logic  Operator=OR  IconShape=distinctive  AllPortsSameDT=off  OutDataTypeStr=boolean
  Relational Operator : RelationalOperator  Operator=>  OutDataTypeStr=boolean  RndMeth=Nearest
  Unit Delay Enabled : simulink_need_slupdate/Unit Delay Enabled  vinit=0.0  tsamp=-1
      settings: SourceProductName=Simulink  SourceProductBaseCode=SL
  Unit Delay Enabled1 : simulink_need_slupdate/Unit Delay Enabled  vinit=0.0  tsamp=-1
      settings: SourceProductName=Simulink  SourceProductBaseCode=SL
  Unit Delay Enabled2 : simulink_need_slupdate/Unit Delay Enabled  vinit=0.0  tsamp=-1
      settings: SourceProductName=Simulink  SourceProductBaseCode=SL
  angleOut : Outport
  validOut : Outport  Port=2
  wires:
  magIn/1 -> Delay5/1
  angleIn/1 -> Delay1/1
  HDL Counter/1 -> Compare To Constant/1
  Compare To Constant/1 -> Unit Delay Enabled2/2, Logical Operator/2, Delay3/1
  Unit Delay Enabled1/1 -> Unit Delay Enabled2/1
  validIn/1 -> Delay2/1
  Delay5/1 -> Relational Operator/1, Unit Delay Enabled/1
  Delay2/1 -> HDL Counter/1
  Unit Delay Enabled2/1 -> angleOut/1
  Delay3/1 -> validOut/1
  Unit Delay Enabled/1 -> Relational Operator/2
  Relational Operator/1 -> Logical Operator/1
  Logical Operator/1 -> Unit Delay Enabled1/2, Unit Delay Enabled/2
  Delay1/1 -> Unit Delay Enabled1/1

== system HDLLTE/LTE_Detector_HDL/Frequency_Estimation/Cyclic_Prefix_Correlator ==
  note: Correlate the signal with itself
      | delayed by the FFT length (128 samples).
  note: Integrate across part of the CP length, which is 9 samples. However we use 8 samples here to optimize for HDL implementation.
  note: Finally average across 7 OFDM symbols, i.e. the number in
      | each slot.
  dataIn : Inport
  Delay1 : Delay  DelayLength=1  InitialCondition=0  UseCircularBuffer=on
  Delay2 : Delay  DelayLength=128  InitialCondition=0
  Delay3 : Delay  DelayLength=1  InitialCondition=0  UseCircularBuffer=on
  Delay5 : Delay  DelayLength=1  InitialCondition=0  UseCircularBuffer=on
  Moving_Average : Subsystem
  Product : Product  OutDataTypeStr=fixdt(1,24,23)  RndMeth=Round
  Slot_Average : Subsystem
  complexConj : Math  Operator=conj  SaturateOnIntegerOverflow=on
  corrOut : Outport
  wires:
  Product/1 -> Delay5/1
  Delay3/1 -> Product/2
  Delay2/1 -> complexConj/1
  Slot_Average/1(dataOut) -> corrOut/1
  Moving_Average/1(dataOut) -> Slot_Average/1(dataIn)
  complexConj/1 -> Delay3/1
  Delay5/1 -> Moving_Average/1(dataIn)
  Delay1/1 -> Product/1
  dataIn/1 -> Delay2/1, Delay1/1

== system HDLLTE/LTE_Detector_HDL/Frequency_Estimation/Rect_to_Polar ==
  dataIn : Inport
  Complex to Magnitude-Angle HDL Optimized : dspmathops/Complex to Magnitude-Angle HDL Optimized  NumIterationsSource=Auto  NumIterations=16  OutputFormat=Magnitude and angle  AngleFormat=Normalized  ScaleOutput=on  SimulateUsing=Code generation
      settings: SourceProductName=DSP System Toolbox  SourceProductBaseCode=DS
  Constant : Constant  OutDataTypeStr=boolean  SampleTime=simParams.TsRx
  Delay1 : Delay  InitialCondition=0  UseCircularBuffer=on
  Delay2 : Delay  DelayLength=1  InitialCondition=0  UseCircularBuffer=on
  Delay3 : Delay  DelayLength=1  InitialCondition=0  UseCircularBuffer=on
  Delay4 : Delay  DelayLength=1  InitialCondition=0  UseCircularBuffer=on
  Delay5 : Delay  InitialCondition=0  UseCircularBuffer=on
  Gain : Gain  Gain=0.5  OutDataTypeStr=fixdt(1,27,27)
  Signal Specification1 : SignalSpecification  Dimensions=1
  magOut : Outport
  angleOut : Outport  Port=2
  validOut : Outport  Port=3
  wires:
  Gain/1 -> angleOut/1
  dataIn/1 -> Signal Specification1/1
  Constant/1 -> Delay1/1
  Delay5/1 -> Complex to Magnitude-Angle HDL Optimized/1
  Delay1/1 -> Complex to Magnitude-Angle HDL Optimized/2
  Delay2/1 -> magOut/1
  Delay3/1 -> Gain/1
  Delay4/1 -> validOut/1
  Complex to Magnitude-Angle HDL Optimized/1 -> Delay2/1
  Complex to Magnitude-Angle HDL Optimized/3 -> Delay4/1
  Complex to Magnitude-Angle HDL Optimized/2 -> Delay3/1
  Signal Specification1/1 -> Delay5/1

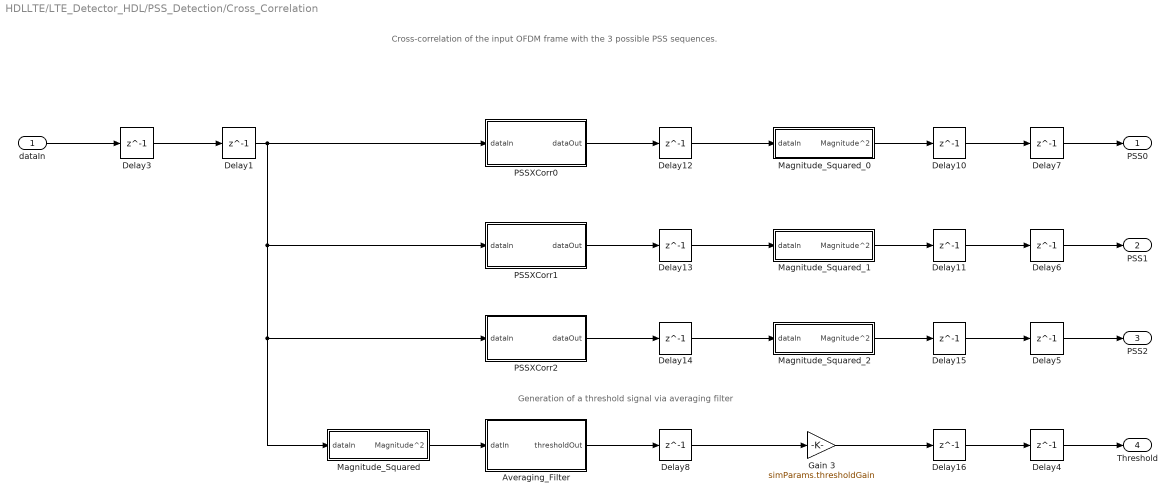
== system HDLLTE/LTE_Detector_HDL/PSS_Detection/Cross_Correlation ==
  note: Cross-correlation of the input OFDM frame with the 3 possible PSS sequences.
  note: Generation of a threshold signal via averaging filter
  dataIn : Inport
  Averaging_Filter : Subsystem
  Delay{1,3..8,10..16} (14 alike) : Delay  DelayLength=1  InitialCondition=0
  Gain 3 : Gain  Gain=simParams.thresholdGain  OutDataTypeStr=fixdt(1,32,20)
  Magnitude_Squared : Subsystem
  Magnitude_Squared_0 : Subsystem
  Magnitude_Squared_1 : Subsystem
  Magnitude_Squared_2 : Subsystem
  PSSXCorr0 : Subsystem  mask(ComplexFIRFilter){PSSIdxZeroBased=0}
      mask prompts: PSSIdxZeroBased "PSS Sequence (0, 1, 2)"
      mask help: Implements a complex valued FIR filter.
      mask init:
      | % convert zero-based index to MATLAB one-based index for accessing matrix
      | PSSIdx = PSSIdxZeroBased + 1;
  PSSXCorr1 : Subsystem  mask(ComplexFIRFilter){PSSIdxZeroBased=1}
      mask prompts: PSSIdxZeroBased "PSS Sequence (0, 1, 2)"
      mask help: Implements a complex valued FIR filter.
      mask init:
      | % convert zero-based index to MATLAB one-based index for accessing matrix
      | PSSIdx = PSSIdxZeroBased + 1;
  PSSXCorr2 : Subsystem  mask(ComplexFIRFilter){PSSIdxZeroBased=2}
      mask prompts: PSSIdxZeroBased "PSS Sequence (0, 1, 2)"
      mask help: Implements a complex valued FIR filter.
      mask init:
      | % convert zero-based index to MATLAB one-based index for accessing matrix
      | PSSIdx = PSSIdxZeroBased + 1;
  PSS0 : Outport
  PSS1 : Outport  Port=2
  PSS2 : Outport  Port=3
  Threshold : Outport  Port=4
  wires:
  dataIn/1 -> Delay3/1
  Delay10/1 -> Delay7/1
  Delay11/1 -> Delay6/1
  Delay15/1 -> Delay5/1
  Delay16/1 -> Delay4/1
  Delay4/1 -> Threshold/1
  Delay5/1 -> PSS2/1
  Delay6/1 -> PSS1/1
  Delay7/1 -> PSS0/1
  Delay3/1 -> Delay1/1
  Delay1/1 -> PSSXCorr1/1(dataIn), PSSXCorr2/1(dataIn), Magnitude_Squared/1(dataIn), PSSXCorr0/1(dataIn)
  Delay12/1 -> Magnitude_Squared_0/1(dataIn)
  PSSXCorr0/1(dataOut) -> Delay12/1
  Magnitude_Squared_0/1(Magnitude^2) -> Delay10/1
  Delay13/1 -> Magnitude_Squared_1/1(dataIn)
  PSSXCorr1/1(dataOut) -> Delay13/1
  Magnitude_Squared_1/1(Magnitude^2) -> Delay11/1
  Delay14/1 -> Magnitude_Squared_2/1(dataIn)
  PSSXCorr2/1(dataOut) -> Delay14/1
  Magnitude_Squared_2/1(Magnitude^2) -> Delay15/1
  Magnitude_Squared/1(Magnitude^2) -> Averaging_Filter/1(datIn)
  Averaging_Filter/1(thresholdOut) -> Delay8/1
  Delay8/1 -> Gain 3/1
  Gain 3/1 -> Delay16/1

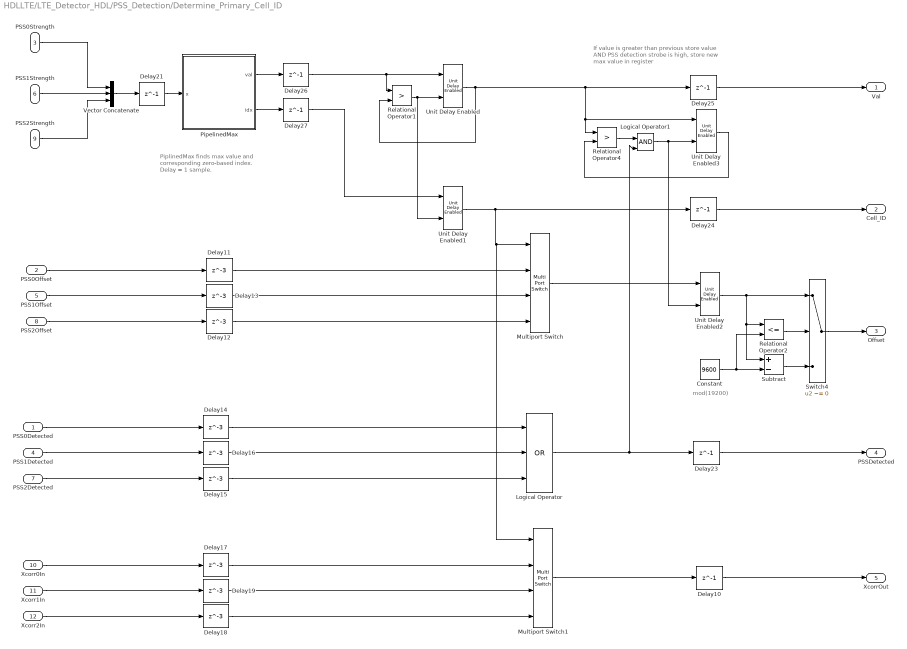
== system HDLLTE/LTE_Detector_HDL/PSS_Detection/Determine_Primary_Cell_ID ==
  note: mod(19200)
  note: If value is greater than previous store value
      | AND PSS detection strobe is high,
      | store new max value in register
  note: PiplinedMax finds max value and
      | corresponding zero-based index.
      | Delay = 1 sample.
  PSS0Detected : Inport
  PSS0Offset : Inport  Port=2
  PSS0Strength : Inport  Port=3
  PSS1Detected : Inport  Port=4
  PSS1Offset : Inport  Port=5
  PSS1Strength : Inport  Port=6
  PSS2Detected : Inport  Port=7
  PSS2Offset : Inport  Port=8
  PSS2Strength : Inport  Port=9
  Xcorr0In : Inport  Port=10
  Xcorr1In : Inport  Port=11
  Xcorr2In : Inport  Port=12
  Constant : Constant  Value=9600  OutDataTypeStr=fixdt(0,14,0)  SampleTime=simParams.TsRx
  Delay{10,21,23..27} (7 alike) : Delay  DelayLength=1  InitialCondition=0  InputProcessing=Columns as channels (frame based)
  Delay{11..19} (9 alike) : Delay  DelayLength=3  InitialCondition=0  InputProcessing=Columns as channels (frame based)
  Logical Operator : Logic  Operator=OR  Inputs=3  IconShape=distinctive  AllPortsSameDT=off  OutDataTypeStr=boolean
  Logical Operator1 : Logic  IconShape=distinctive  AllPortsSameDT=off  OutDataTypeStr=boolean
  Multiport Switch : MultiPortSwitch  DataPortOrder=Zero-based contiguous
  Multiport Switch1 : MultiPortSwitch  DataPortOrder=Zero-based contiguous
  PipelinedMax : MATLAB Function  TreatAsAtomicUnit=on
  Relational Operator1 : RelationalOperator  Operator=>  OutDataTypeStr=boolean  RndMeth=Nearest
  Relational Operator2 : RelationalOperator  Operator=<=  OutDataTypeStr=boolean  RndMeth=Nearest
  Relational Operator4 : RelationalOperator  Operator=>  OutDataTypeStr=boolean  RndMeth=Nearest
  Subtract : Sum  Inputs=+-  RndMeth=Round
  Switch4 : Switch  Criteria=u2 ~= 0  Threshold=384  OutDataTypeStr=Inherit: Inherit via back propagation
  Unit Delay Enabled{,1..3} (4 alike) : simulink_need_slupdate/Unit Delay Enabled  vinit=0.0  tsamp=-1
      settings: SourceProductName=Simulink  SourceProductBaseCode=SL
  Vector Concatenate : Concatenate  NumInputs=3  Mode=Multidimensional array  ConcatenateDimension=2
  Val : Outport
  Cell_ID : Outport  Port=2
  "Offset " : Outport  Port=3
  PSSDetected : Outport  Port=4
  XcorrOut : Outport  Port=5
  wires:
  PSS0Strength/1 -> Vector Concatenate/1
  Relational Operator1/1 -> Unit Delay Enabled1/2, Unit Delay Enabled/2
  PSS2Strength/1 -> Vector Concatenate/3
  Unit Delay Enabled1/1 -> Multiport Switch1/1, Multiport Switch/1, Delay24/1
  PSS2Detected/1 -> Delay15/1
  PSS0Offset/1 -> Delay11/1
  PSS1Offset/1 -> Delay13/1
  PSS2Offset/1 -> Delay12/1
  PSS0Detected/1 -> Delay14/1
  PSS1Detected/1 -> Delay16/1
  Unit Delay Enabled/1 -> Relational Operator1/2, Delay25/1, Unit Delay Enabled3/1, Relational Operator4/1
  Unit Delay Enabled3/1 -> Relational Operator4/2
  Multiport Switch/1 -> Unit Delay Enabled2/1
  Logical Operator/1 -> Logical Operator1/2, Delay23/1
  Logical Operator1/1 -> Unit Delay Enabled2/2, Unit Delay Enabled3/2
  Relational Operator4/1 -> Logical Operator1/1
  Relational Operator2/1 -> Switch4/2
  Unit Delay Enabled2/1 -> Subtract/1, Relational Operator2/1, Switch4/1
  Constant/1 -> Relational Operator2/2, Subtract/2
  Switch4/1 -> "Offset "/1
  Subtract/1 -> Switch4/3
  Multiport Switch1/1 -> Delay10/1
  Xcorr0In/1 -> Delay17/1
  Xcorr1In/1 -> Delay19/1
  Xcorr2In/1 -> Delay18/1
  Delay10/1 -> XcorrOut/1
  PSS1Strength/1 -> Vector Concatenate/2
  Delay23/1 -> PSSDetected/1
  Delay24/1 -> Cell_ID/1
  Delay25/1 -> Val/1
  PipelinedMax/2(idx) -> Delay27/1
  Delay26/1 -> Relational Operator1/1, Unit Delay Enabled/1
  Delay27/1 -> Unit Delay Enabled1/1
  Vector Concatenate/1 -> Delay21/1
  PipelinedMax/1(val) -> Delay26/1
  Delay11/1 -> Multiport Switch/2
  Delay13/1 -> Multiport Switch/3
  Delay15/1 -> Logical Operator/3
  Delay16/1 -> Logical Operator/2
  Delay14/1 -> Logical Operator/1
  Delay12/1 -> Multiport Switch/4
  Delay17/1 -> Multiport Switch1/2
  Delay19/1 -> Multiport Switch1/3
  Delay18/1 -> Multiport Switch1/4
  Delay21/1 -> PipelinedMax/1(x)
